simulink model "LCK_DanishV01"  (R2018b)
settings: Solver=FixedStepDiscrete  StartTime=0.0  StopTime=inf  FixedStep=0.01  RelTol=1e-3
PostLoadFcn:
  | if any(exist('dsrtsu_mdlpostloadfcn', 'file') ~= 0), dsrtsu_mdlpostloadfcn('Execute', bdroot); end
values from neighbouring files (symbols this model uses):
  C_DEG2RAD = 0.0175    [LCK_Macro.sldd]
  C_KPH2MPS = 0.2778    [LCK_Macro.sldd]
  C_NEARZERO = 0.0001    [LCK_Macro.sldd]
  C_ONE = 1.0    [LCK_Macro.sldd]
  C_RAD2DEG = 57.2958    [LCK_Macro.sldd]
  C_ZERO = 0.0    [LCK_Macro.sldd]
  k_accel_pedal_pos_per_speed_x : value not decoded    [LCK_LogicPara.sldd]
  k_accel_pedal_pos_per_speed_z : value not decoded    [LCK_LogicPara.sldd]
  k_brake_suprress_hold = 1000.0    [LCK_LogicPara.sldd]
  k_driver_appl_torque_filt = 50.0    [LCK_LogicPara.sldd]
  k_driver_suppression_hold_time = 3000.0    [LCK_LogicPara.sldd]
  k_hands_on_wheel_hold_msec = 500.0    [LCK_LogicPara.sldd]
  k_hands_on_wheel_torque_hi = 0.2    [LCK_LogicPara.sldd]
  k_hands_on_wheel_torque_lo = 0.15    [LCK_LogicPara.sldd]
  k_handsoff_delay_cycles = 50.0    [LCK_LogicPara.sldd]
  k_handsoff_torq_Lo_CR = 0.3    [LCK_LogicPara.sldd]
  k_handson_delay_cycles = 5.0    [LCK_LogicPara.sldd]
  k_HighAccel_suppress_hold = 3000.0    [LCK_LogicPara.sldd]
  k_HLR_suprress_hold = 3000.0    [LCK_LogicPara.sldd]
  k_hs_StrAng_CR_threshold_z : value not decoded    [LCK_LogicPara.sldd]
  k_LC_Exit_Switch = 0.0    [LCK_LogicPara.sldd]
  k_LCG_Configured = 1.0    [LCK_LogicPara.sldd]
  k_LCK_A0_Rdy2Act_UseConst = 0.0    [LCK_LogicPara.sldd]
  k_LCK_A0Fac_ActSta : value not decoded    [LCK_CtrlPara.sldd]
  k_LCK_A0Fac_DrvStm : value not decoded    [LCK_CtrlPara.sldd]
  k_LCK_A0Shift_LftCurv : value not decoded    [LCK_CtrlPara.sldd]
  k_LCK_A0Shift_RgtCurv : value not decoded    [LCK_CtrlPara.sldd]
  k_LCK_A0Shift_StraLan = 0.0    [LCK_CtrlPara.sldd]
  k_LCK_A0ShiftFac_Dy_LftCurv : value not decoded    [LCK_CtrlPara.sldd]
  k_LCK_A0ShiftFac_Dy_RgtCurv : value not decoded    [LCK_CtrlPara.sldd]
  k_LCK_A0ShiftFac_Vspd : value not decoded    [LCK_CtrlPara.sldd]
  k_LCK_accel_inhibit_thold = 35.0    [LCK_LogicPara.sldd]
  k_LCK_Active2Ready_Mask = 255.0    [LCK_LogicPara.sldd]
  k_LCK_CvatRateBks : value not decoded    [LCK_CtrlPara.sldd]
  k_LCK_CvatrBks : value not decoded    [LCK_CtrlPara.sldd]
  k_LCK_DFac_Dy : value not decoded    [LCK_CtrlPara.sldd]
  k_LCK_DFac_Dy_Curv : value not decoded    [LCK_CtrlPara.sldd]
  k_LCK_DFac_HaCurCen : value not decoded    [LCK_CtrlPara.sldd]
  k_LCK_DFac_HaCurSid : value not decoded    [LCK_CtrlPara.sldd]
  k_LCK_DFac_HadCurCen : value not decoded    [LCK_CtrlPara.sldd]
  k_LCK_DFac_HadCurSid : value not decoded    [LCK_CtrlPara.sldd]
  k_LCK_DFac_HadStrCen : value not decoded    [LCK_CtrlPara.sldd]
  k_LCK_DFac_HadStrSid : value not decoded    [LCK_CtrlPara.sldd]
  k_LCK_DFac_HaStrCen : value not decoded    [LCK_CtrlPara.sldd]
  k_LCK_DFac_HaStrSid : value not decoded    [LCK_CtrlPara.sldd]
  k_LCK_DFac_Rad : value not decoded    [LCK_CtrlPara.sldd]
  k_LCK_DFac_SA_CurCen : value not decoded    [LCK_CtrlPara.sldd]
  k_LCK_DFac_SA_CurSid : value not decoded    [LCK_CtrlPara.sldd]
  k_LCK_DFac_SA_StrCen : value not decoded    [LCK_CtrlPara.sldd]
  k_LCK_DFac_SA_StrSid : value not decoded    [LCK_CtrlPara.sldd]
  k_LCK_DFac_SS_CurCen : value not decoded    [LCK_CtrlPara.sldd]
  k_LCK_DFac_SS_CurSid : value not decoded    [LCK_CtrlPara.sldd]
  k_LCK_DFac_SS_StrCen : value not decoded    [LCK_CtrlPara.sldd]
  k_LCK_DFac_SS_StrSid : value not decoded    [LCK_CtrlPara.sldd]
  k_LCK_DFac_Vspd : value not decoded    [LCK_CtrlPara.sldd]
  k_LCK_DlyTm_DrvStim = 0.2    [LCK_CtrlPara.sldd]
  k_LCK_DTermMax = 2.0    [LCK_CtrlPara.sldd]
  k_LCK_DyBks_Curv : value not decoded    [LCK_CtrlPara.sldd]
  k_LCK_Enable_POOnly = 1.0    [LCK_LogicPara.sldd]
  k_LCK_Entry_DistBuffer = 0.1    [LCK_LogicPara.sldd]
  k_LCK_Fac_Vspd2RngThr_FalRec = 0.23    [LCK_CtrlPara.sldd]
  k_LCK_Ffw_CvatSwh = 0.0    [LCK_CtrlPara.sldd]
  k_LCK_Ffw_DyBks : value not decoded    [LCK_CtrlPara.sldd]
  k_LCK_Ffw_TimCon_CmdFlt = 0.0    [LCK_CtrlPara.sldd]
  k_LCK_FfwDeltaFac_Rad_Lft : value not decoded    [LCK_CtrlPara.sldd]
  k_LCK_FfwDeltaFac_Rad_Rgt : value not decoded    [LCK_CtrlPara.sldd]
  k_LCK_FfwDeltaFac_Vspd : value not decoded    [LCK_CtrlPara.sldd]
  k_LCK_FfwFac_CvatRate_Lft : value not decoded    [LCK_CtrlPara.sldd]
  k_LCK_FfwFac_CvatRate_Rgt : value not decoded    [LCK_CtrlPara.sldd]
  k_LCK_FfwFac_Dy : value not decoded    [LCK_CtrlPara.sldd]
  k_LCK_FfwFac_Rad_Lft : value not decoded    [LCK_CtrlPara.sldd]
  k_LCK_FfwFac_Rad_Rgt : value not decoded    [LCK_CtrlPara.sldd]
  k_LCK_FfwFac_Vspd : value not decoded    [LCK_CtrlPara.sldd]
  k_LCK_FfwTorq_Cvat : value not decoded    [LCK_CtrlPara.sldd]
  k_LCK_HAFac_ActSta : value not decoded    [LCK_CtrlPara.sldd]
  k_LCK_HAFac_DrvStm : value not decoded    [LCK_CtrlPara.sldd]
  k_LCK_HaloTime = 2000.0    [LCK_LogicPara.sldd]
  k_LCK_HaloTime_Switch = 0.0    [LCK_LogicPara.sldd]
  k_LCK_HARFac_ActSta : value not decoded    [LCK_CtrlPara.sldd]
  k_LCK_HARFac_DrvStm : value not decoded    [LCK_CtrlPara.sldd]
  k_LCK_Hed_DyBks : value not decoded    [LCK_CtrlPara.sldd]
  k_LCK_HedAngDiffX : value not decoded    [LCK_CtrlPara.sldd]
  k_LCK_HedAngRateDiffX : value not decoded    [LCK_CtrlPara.sldd]
  k_LCK_HndsOnWhel_DlyTm_Idl2Rdy = 0.0    [LCK_LogicPara.sldd]
  k_LCK_host_veh_width = 1.86    [LCK_LogicPara.sldd]
  k_LCK_Idle2Ready_Mask = 239.0    [LCK_LogicPara.sldd]
  k_LCK_Junc_SusTime = 1.0    [LCK_LogicPara.sldd]
  k_LCK_KpKdDecSlopeLmt = 10.0    [LCK_CtrlPara.sldd]
  k_LCK_KpKdIncSlopeLmt = 5.0    [LCK_CtrlPara.sldd]
  k_LCK_Lat_Ctrl_DFac_Lft = 1.0    [LCK_CtrlPara.sldd]
  k_LCK_Lat_Ctrl_DFac_Rgt = 1.05    [LCK_CtrlPara.sldd]
  k_LCK_Lat_Ctrl_Kd = 0.8    [LCK_CtrlPara.sldd]
  k_LCK_Lat_Ctrl_Ki = 0.5    [LCK_CtrlPara.sldd]
  k_LCK_Lat_Ctrl_Kp = 0.7    [LCK_CtrlPara.sldd]
  k_LCK_Lat_Ctrl_Kp_NearGain = 0.7    [LCK_CtrlPara.sldd]
  k_LCK_Lat_Ctrl_PFac_Lft = 1.0    [LCK_CtrlPara.sldd]
  k_LCK_Lat_Ctrl_PFac_Rgt = 1.05    [LCK_CtrlPara.sldd]
  k_LCK_Lat_Ctrl_TimCon_CmdFlt = 5.0    [LCK_CtrlPara.sldd]
  k_LCK_Lat_DFac_Rad : value not decoded    [LCK_CtrlPara.sldd]
  k_LCK_Lat_DFac_SS_Cur : value not decoded    [LCK_CtrlPara.sldd]
  k_LCK_Lat_DFac_SS_Str : value not decoded    [LCK_CtrlPara.sldd]
  k_LCK_Lat_DFac_Vspd : value not decoded    [LCK_CtrlPara.sldd]
  k_LCK_Lat_DyBks : value not decoded    [LCK_CtrlPara.sldd]
  k_LCK_Lat_IFac_Rad : value not decoded    [LCK_CtrlPara.sldd]
  k_LCK_Lat_IFac_Vspd : value not decoded    [LCK_CtrlPara.sldd]
  k_LCK_Lat_ILmtFac_Dy_CurvLan : value not decoded    [LCK_CtrlPara.sldd]
  k_LCK_Lat_ILmtFac_Dy_StraLan : value not decoded    [LCK_CtrlPara.sldd]
  k_LCK_Lat_ILmtFac_Rad : value not decoded    [LCK_CtrlPara.sldd]
  k_LCK_Lat_ILmtFac_Rad_NearGain = 1.0    [LCK_CtrlPara.sldd]
  k_LCK_Lat_ILmtFac_Vspd_CurvLan : value not decoded    [LCK_CtrlPara.sldd]
  k_LCK_Lat_ILmtFac_Vspd_StraLan : value not decoded    [LCK_CtrlPara.sldd]
  k_LCK_Lat_ITermLmt_Dy = 1.0    [LCK_CtrlPara.sldd]
  k_LCK_Lat_KpKdDecSlopeLmt = 10.0    [LCK_CtrlPara.sldd]
  k_LCK_Lat_KpKdIncSlopeLmt = 10.0    [LCK_CtrlPara.sldd]
  k_LCK_Lat_PFac_Dy_InnLftCur : value not decoded    [LCK_CtrlPara.sldd]
  k_LCK_Lat_PFac_Dy_InnRgtCur : value not decoded    [LCK_CtrlPara.sldd]
  k_LCK_Lat_PFac_Dy_OutLftCur : value not decoded    [LCK_CtrlPara.sldd]
  k_LCK_Lat_PFac_Dy_OutRgtCur : value not decoded    [LCK_CtrlPara.sldd]
  k_LCK_Lat_PFac_Dy_Str : value not decoded    [LCK_CtrlPara.sldd]
  k_LCK_Lat_PFac_Rad : value not decoded    [LCK_CtrlPara.sldd]
  ... (+153 more)
undefined symbols (not defined in the file or in its folder): k_LCK_CurvBks, K_LCK_SPA0A1A2_LMRngCmp_y
libraries: LateralControl_fcns_lib x58, simulink x24
(part 46 of 47)

== stateflow chart LCK_DanishV01/Lateral_Control_Module/LCK_State_Ctrl/LCK_Mode_Transition/Det_TJA_Lat_Req/Chart ==
  state TJA_Lat_Req_Reset
    en:
    TJA_Lat_Req=0;
  state TJA_Lat_Req_Set
    en:
    TJA_Lat_Req=1;
  (default) -> TJA_Lat_Req_Reset
  TJA_Lat_Req_Reset -> TJA_Lat_Req_Set : [TJA_State == 3]
  TJA_Lat_Req_Set -> TJA_Lat_Req_Reset : [TJA_State < 3 || TJA_State == 5]
  data: TJA_State input; TJA_Lat_Req output double

== stateflow chart LCK_DanishV01/Lateral_Control_Module/Lat_HMI/Trigger Hold Counter/Trigger Hold ==
  settings: description=_GWMH9P5.LCK.111_13_
  (default) -> (junction 11)
  (junction 11) -> (junction 13) [order 1] : [(Trigger==1)]...
      | {count = 0;}
  (junction 11) -> (junction 14) [order 2]
  (junction 13) -> (junction 17)
  (junction 14) -> (junction 17) [order 1] : [count<= hold_time]
  (junction 14) -> (junction 15) [order 2] : {Out = 0;}
  (junction 17) -> (junction 16) : {
      | Out = 1;...
      | count = count + ML_TIME_MSEC;
      | }
  (junction 15) -> (junction 16)
  (junction 16) -> (junction 25)
  data: Trigger input [0..1]; hold_time input; Out output boolean [0..1]; count output single; ML_TIME_MSEC parameter single
  data Trigger settings: description=_GWMH9P5.LCK.111_116_
  data hold_time settings: description=_GWMH9P5.LCK.111_117_
  data Out settings: description=|
      | _GACA26P4.LCK.111_66_
      | $TL$ type=Bool; date=20190416T145812; $TL$
  data count settings: description=|
      | _GACA26P4.LCK.111_67_
      | $TL$ type=Float32; date=20190416T145816; $TL$
  data ML_TIME_MSEC settings: description=|
      | _GACA26P4.LCK.111_68_
      | $TL$ name=$O; type=ESR_Typedefs/unsigned8_T; class=EXTERN_MACRO; date=20190416T150613; $TL$

== stateflow chart LCK_DanishV01/Lateral_Control_Module/LC_Path_Process/Chart1 ==
  state LC_Phase1
    en:
    LC_A0 = SPP_A0 - Path_Palnning_Lat_Offset ;
    du:
    LC_A0 = SPP_A0 - Path_Palnning_Lat_Offset;
  state LC_Phase3
    en:
    LC_A0 = SPP_A0 - Path_Palnning_Lat_Offset;
    du:
    LC_A0 = SPP_A0 - Path_Palnning_Lat_Offset;
  state LC_Phase4
    en:
    LC_A0 = SPP_A0 - Path_Palnning_Lat_Offset;
    du:
    LC_A0 = SPP_A0 - Path_Palnning_Lat_Offset;
  state LC_Phase2
    en:
    LC_A0 = SPP_A0 - Path_Palnning_Lat_Offset;
    du:
    LC_A0 = SPP_A0 - Path_Palnning_Lat_Offset;
  state Initialization
    en:
    LC_A0 = 0;
  state LC_Phase3p5
    en:
    LC_A0 = SPP_A0 - Lane_Width-Path_Palnning_Lat_Offset;
    du:
    LC_A0 = SPP_A0 - Lane_Width-Path_Palnning_Lat_Offset;
  state LC_Phase1p5
    en:
    LC_A0 = SPP_A0 + Lane_Width - Path_Palnning_Lat_Offset;
    du:
    LC_A0 = SPP_A0 + Lane_Width - Path_Palnning_Lat_Offset;
  Initialization -> LC_Phase3 [order 2] : [LC_Phase == 3]
  Initialization -> LC_Phase1 [order 1] : [LC_Phase == 1]
  LC_Phase3 -> Initialization [order 1] : [LC_Phase == 0]
  LC_Phase1 -> Initialization [order 1] : [LC_Phase == 0]
  LC_Phase4 -> LC_Phase3 [order 1] : [LC_Phase == 3]
  LC_Phase3 -> LC_Phase4 [order 3] : [(LC_Phase == 4)&&(LC_path_gen_flag==1)]
  LC_Phase3p5 -> LC_Phase3 [order 2] : [LC_Phase == 3]
  LC_Phase3 -> LC_Phase3p5 [order 2] : [(LC_Phase == 4)&&(LC_path_gen_flag==0)]
  LC_Phase1 -> LC_Phase1p5 [order 2] : [(LC_Phase == 2)&&(LC_path_gen_flag==0)]
  LC_Phase1p5 -> LC_Phase1 [order 2] : [LC_Phase == 1]
  LC_Phase1 -> LC_Phase2 [order 3] : [(LC_Phase == 2)&&(LC_path_gen_flag==1)]
  LC_Phase2 -> LC_Phase1 [order 1] : [LC_Phase == 1]
  LC_Phase4 -> Initialization [order 2] : [LC_Phase == 0]
  LC_Phase3p5 -> LC_Phase4 [order 3] : [LC_path_gen_flag==1]
  LC_Phase1p5 -> LC_Phase2 [order 3] : [LC_path_gen_flag==1]
  LC_Phase2 -> Initialization [order 2] : [LC_Phase == 0]
  (default) -> Initialization
  LC_Phase3p5 -> Initialization [order 1] : [LC_Phase == 0]
  LC_Phase1p5 -> Initialization [order 1] : [LC_Phase == 0]
  data: LC_Phase input; SPP_A0 input; LC_A0 output single; Lane_Width input; Path_Palnning_Lat_Offset input; LC_path_gen_flag input

== stateflow chart LCK_DanishV01/Lateral_Control_Module/Adas_Lateral_Control_LCK_Core/Module 6/Determination Of Cen Flag/Chart ==
  state State_0
    entry:Cen_Flag =LCK_BOOLEAN_TURE;
  state State_1
    entry:Cen_Flag =LCK_BOOLEAN_FALSE;
  (default) -> (junction 6)
  (junction 6) -> State_1 [order 2]
  (junction 6) -> State_0 [order 1] : [Dy<CenLowLmt]
  State_0 -> State_1 : [Dy>=CenUpLmt]
  State_1 -> State_0 : [Dy<=CenLowLmt]
  data: Dy input; CenUpLmt input; CenLowLmt input; Cen_Flag output boolean; LCK_BOOLEAN_TURE parameter; LCK_BOOLEAN_FALSE parameter

== stateflow chart LCK_DanishV01/Lateral_Control_Module/Adas_Lateral_Control_LCK_Core/Module 6/Determination of Str Flag/Chart1 ==
  state State_0
    entry:Str_Flag =LCK_BOOLEAN_TURE;
  state State_1
    entry:Str_Flag =LCK_BOOLEAN_TURE;
  (default) -> (junction 6)
  (junction 6) -> State_1 [order 2]
  (junction 6) -> State_0 [order 1] : [Radius>RadiusUpLmt]
  State_0 -> State_1 : [Radius<=RadiusLowLmt]
  State_1 -> State_0 : [Radius>RadiusUpLmt]
  data: Radius input; RadiusUpLmt input; RadiusLowLmt input; Str_Flag output boolean; LCK_BOOLEAN_TURE parameter boolean; LCK_BOOLEAN_FALSE parameter boolean

== stateflow chart LCK_DanishV01/Lateral_Control_Module/LCK_State_Ctrl/LCK_Mode_Transition/Determination_of_Lat_Ctrl_Req/LCK_TJA_LatRq_Manager ==
  state LatRqOn
    state TJA_Rq
      en:
      LatRq=1;
      LCKON_TJAOFF=0;
    state LCK_Rq
      en:
      LatRq=1;
      LCKON_TJAOFF=1;
    TJA_Rq -> LCK_Rq [order 1] : [TJA_LatCtrl_Rq==0 && ...
        | LCK_Switch==1 && ...
        | VehicleSpd>=k_LCK_TJALCK_SWSpeed]
    LCK_Rq -> TJA_Rq [order 2] : [TJA_LatCtrl_Rq==1]
  state LatRqOff
    en:LatRq=0;
    LCKON_TJAOFF=0;
  LCK_Rq -> LatRqOff [order 1] : [LCK_Switch==0 ||...
      |  VehicleSpd<(k_LCK_TJALCK_SWSpeed-5)]
  LatRqOff -> LCK_Rq [order 2] : [LCK_Switch==1 &&...
      |  VehicleSpd>=k_LCK_TJALCK_SWSpeed]
  LatRqOff -> TJA_Rq [order 1] : [TJA_LatCtrl_Rq==1]
  TJA_Rq -> LatRqOff [order 2] : [TJA_LatCtrl_Rq==0]
  (default) -> LatRqOff
  data: LCKON_TJAOFF output; LatRq output; TJA_LatCtrl_Rq input; LCK_Switch input; VehicleSpd input; k_LCK_TJALCK_SWSpeed input

== stateflow chart LCK_DanishV01/Lateral_Control_Module/LCK_State_Ctrl/LCK_Mode_Transition/READY2ACTIVE_Magic_Claculation/Trigger Hold2/Trigger Hold ==
  settings: description=_GWMH9P5.LCK.111_10_
  (default) -> (junction 11)
  (junction 11) -> (junction 13) [order 1] : [(Trigger==1)]...
      | {count = 0; count_enable=1;}
  (junction 11) -> (junction 14) [order 2]
  (junction 13) -> (junction 17)
  (junction 14) -> (junction 17) [order 1] : [count<= hold_time && count_enable==1 ]
  (junction 14) -> (junction 15) [order 2] : {Out = 0;count_enable=0;}
  (junction 17) -> (junction 16) : {
      | Out = 1;...
      | count = count + ML_TIME_MSEC;
      | }
  (junction 15) -> (junction 16)
  (junction 16) -> (junction 25)
  data: Trigger input [0..1]; hold_time input; Out output single [0..1]; count local single; ML_TIME_MSEC parameter single; count_enable local single
  data Trigger settings: description=_GWMH9P5.LCK.111_109_
  data hold_time settings: description=_GWMH9P5.LCK.111_110_
  data Out settings: description=|
      | _GWMH9P4.LCK.111_134_
      | $TL$ type=Bool; $TL$
  data count settings: description=|
      | _GWMH9P4.LCK.111_130_
      | $TL$ type=UInt32; $TL$
  data ML_TIME_MSEC settings: description=|
      | _GWMH9P4.LCK.111_135_
      | $TL$ name=$O; type=ESR_Typedefs/unsigned8_T; class=EXTERN_MACRO; date=20190206T154634; $TL$
  data count_enable settings: description=|
      | _GWMH9P4.LCK.111_131_
      | $TL$ type=Bool; $TL$

== stateflow chart LCK_DanishV01/Lateral_Control_Module/LCK_State_Ctrl/Det_Driver_Operation/Det_Driver_Steer_Override/Right_distance_sustain_period ==
  settings: description=_GWMH9P5.LCK.111_2_
  note: ML_TIME_MSEC = 10ms
  state Input_Standby
    en:
    sustain_value_out = 0;
    i = 0;
    du:
    sustain_value_out = 0;
    settings: description=_GWMH9P5.LCK.111_30_
  state Output_Message
    du:
    sustain_value_out = 0;
    i = i + ML_TIME_MSEC;
    settings: description=_GWMH9P5.LCK.111_31_
  state Output_Message1
    du:
    sustain_value_out = 1;
    settings: description=_GWMH9P5.LCK.111_32_
  (default) -> Input_Standby
  Input_Standby -> Output_Message : [current_input > 0]
  Output_Message -> Input_Standby [order 2] : [(i < k_override_torq_sustain_period) ...
      | && ( current_input == 0)]
  Output_Message1 -> Input_Standby : [current_input == 0 ]
  Output_Message -> Output_Message1 [order 1] : [(i >=k_override_torq_sustain_period) ...
      | && current_input > 0]
  data: current_input input; i local single; ML_TIME_MSEC parameter single [0..255]; sustain_value_out output single; k_override_torq_sustain_period input; LCK_Mode input
  data current_input settings: description=_GWMH9P5.LCK.111_91_
  data i settings: description=_GWMAB30P2.LCK.111_263_$TL$ type=UInt32; $TL$
  data ML_TIME_MSEC settings: description=|
      | _GWMAB30P2.LCK.111_264_
      | $TL$ name=$O; type=ESR_Typedefs/unsigned8_T; class=EXTERN_MACRO; $TL$
  data sustain_value_out settings: description=_GWMAB30P2.LCK.111_265_$TL$ type=Bool; $TL$
  data k_override_torq_sustain_period settings: description=_GWMH9P5.LCK.111_92_
  data LCK_Mode settings: description=_GWMH9P5.LCK.111_93_

== stateflow chart LCK_DanishV01/Lateral_Control_Module/LCK_State_Ctrl/Det_Driver_Operation/Det_Driver_Steer_Override/left_distance_sustain_period ==
  settings: description=_GWMH9P5.LCK.111_3_
  note: ML_TIME_MSEC = 10ms
  state Input_Standby
    en:
    sustain_value_out = 0;
    i = 0;
    du:
    sustain_value_out = 0;
    settings: description=_GWMH9P5.LCK.111_33_
  state Output_Message
    du:
    sustain_value_out = 0;
    i = i + ML_TIME_MSEC;
    settings: description=_GWMH9P5.LCK.111_34_
  state Output_Message1
    du:
    sustain_value_out = 1;
    settings: description=_GWMH9P5.LCK.111_35_
  (default) -> Input_Standby
  Input_Standby -> Output_Message : [current_input > 0 ]
  Output_Message -> Input_Standby [order 2] : [(i < k_override_torq_sustain_period) ...
      | && ( current_input == 0) ...
      | ]
  Output_Message1 -> Input_Standby : [current_input == 0 ]
  Output_Message -> Output_Message1 [order 1] : [(i >=k_override_torq_sustain_period) ...
      | && current_input > 0]
  data: current_input input; i local single; ML_TIME_MSEC parameter single [0..255]; sustain_value_out output single; k_override_torq_sustain_period input; LCK_Mode input
  data current_input settings: description=_GWMH9P5.LCK.111_94_
  data i settings: description=_GWMAB30P2.LCK.111_268_$TL$ type=UInt32; $TL$
  data ML_TIME_MSEC settings: description=|
      | _GWMAB30P2.LCK.111_269_
      | $TL$ name=$O; type=ESR_Typedefs/unsigned8_T; class=EXTERN_MACRO; $TL$
  data sustain_value_out settings: description=_GWMAB30P2.LCK.111_270_$TL$ type=Bool; $TL$
  data k_override_torq_sustain_period settings: description=_GWMH9P5.LCK.111_95_
  data LCK_Mode settings: description=_GWMH9P5.LCK.111_96_
